simulink model "Discrete_Digital_Analog_Filters"  (R2018a)
settings: Solver=VariableStepAuto  StartTime=0.0  StopTime=1  RelTol=1e-3
libraries: dsparch4 x2
settings Model: Creator=ashwin  LastModifiedBy=ashwin

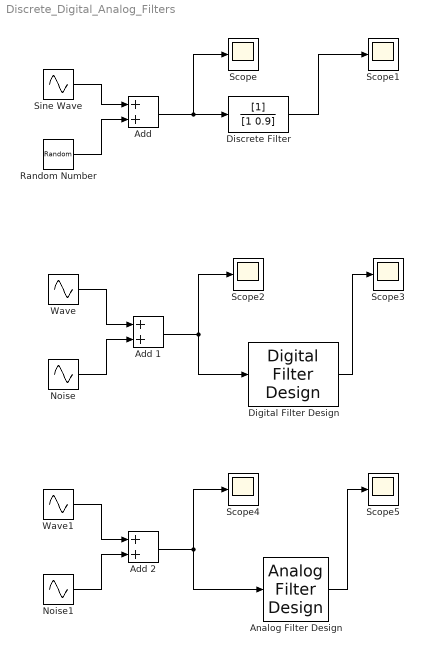
== system Discrete_Digital_Analog_Filters ==
  "Add " : Sum
  Add 1 : Sum
  Add 2 : Sum
  "Analog Filter Design " : dsparch4/Analog Filter Design  method=Butterworth  filttype=Bandpass  N=8  Wlo=100  Whi=80  Rp=2  Rs=40
  "Digital Filter Design " : dsparch4/Digital Filter Design  mwdsp_browser_bugfix_var=off
  "Discrete Filter " : DiscreteFilter  Denominator=[1 0.9]
  Noise : Sin  Amplitude=0.5  Frequency=2*pi*180  SampleTime=1/500
  Noise1 : Sin  Amplitude=0.5  Frequency=2*pi*180  SampleTime=0
  "Random Number " : RandomNumber  Variance=0.1  Seed=777  SampleTime=0.001
  Scope{,1..5} (6 alike) : Scope
  "Sine Wave " : Sin  Frequency=2*pi*5  SampleTime=0.001
  Wave : Sin  Amplitude=2  Frequency=2*pi*10  SampleTime=1/500
  Wave1 : Sin  Amplitude=2  Frequency=2*pi*10  SampleTime=0
  wires:
  "Sine Wave "/1 -> "Add "/1
  "Random Number "/1 -> "Add "/2
  "Add "/1 -> "Discrete Filter "/1, Scope/1
  "Discrete Filter "/1 -> Scope1/1
  Noise/1 -> Add 1/2
  Wave/1 -> Add 1/1
  "Digital Filter Design "/1 -> Scope3/1
  Add 1/1 -> "Digital Filter Design "/1, Scope2/1
  Noise1/1 -> Add 2/2
  "Analog Filter Design "/1 -> Scope5/1
  Wave1/1 -> Add 2/1
  Add 2/1 -> "Analog Filter Design "/1, Scope4/1
